simulink model "convert"  (R2016a)
settings: Solver=VariableStepAuto  StartTime=0.0  StopTime=10.0  RelTol=1e-3
values from neighbouring files (symbols this model uses):
  dt = 0.005    [main.m]
settings Model: Creator=Geraldo  LastModifiedBy=Geraldo

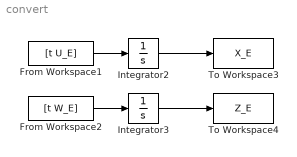
== system convert ==
  From Workspace1 : FromWorkspace  VariableName=[t U_E]  SampleTime=dt
  From Workspace2 : FromWorkspace  VariableName=[t W_E]  SampleTime=dt
  Integrator2 : Integrator
  Integrator3 : Integrator
  To Workspace3 : ToWorkspace  VariableName=X_E  SampleTime=dt
  To Workspace4 : ToWorkspace  VariableName=Z_E  SampleTime=dt
  wires:
  Integrator3/1 -> To Workspace4/1
  Integrator2/1 -> To Workspace3/1
  From Workspace1/1 -> Integrator2/1
  From Workspace2/1 -> Integrator3/1
